simulink model "RCkolo"  (R2015a)
settings: Solver=ode45  StartTime=0.0  StopTime=0.1  MaxStep=10e-6  RelTol=1e-3
values from neighbouring files (symbols this model uses):
  C = 1000e-6    (= 0.001)    [MfajlRCkolo.m]
  R = 5    [MfajlRCkolo.m]
  V = 15    [MfajlRCkolo.m]
libraries: powerlib x6
settings Model: Creator=BLAGI  LastModifiedBy=BLAGI

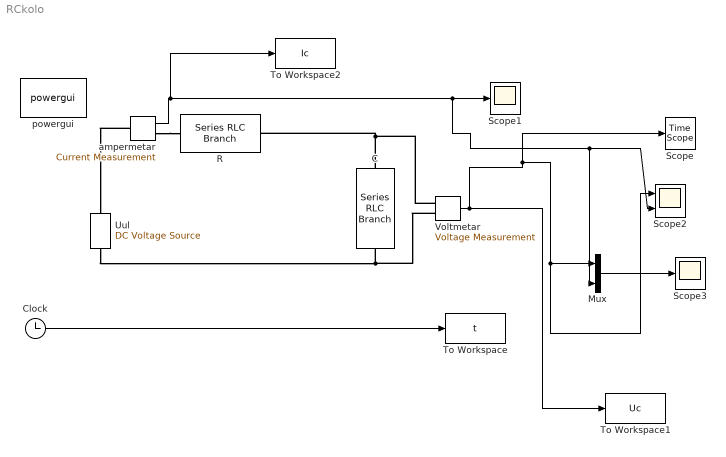
== system RCkolo ==
  C : powerlib/Elements/Series RLC Branch  LConnTagsString=__new0  RConnTagsString=__new0  BranchType=C  Resistance=5  Inductance=1e-3  SetiL0=off  InitialCurrent=0  Capacitance=C  Setx0=on  InitialVoltage=0  Measurements=None
  Clock : Clock
  Mux : Mux  Inputs=2
  R : powerlib/Elements/Series RLC Branch  LConnTagsString=__new0  RConnTagsString=__new0  BranchType=R  Resistance=R  Inductance=1e-3  SetiL0=off  InitialCurrent=0  Capacitance=1e-6  Setx0=off  InitialVoltage=0  Measurements=None
  Scope : TimeScope
  Scope1 : Scope
  Scope2 : Scope  NumInputPorts=2
      settings: YMin=-5~-5  YMax=5~5  SaveName=ScopeData2
  Scope3 : Scope
      settings: SaveName=ScopeData3
  To Workspace : ToWorkspace  VariableName=t  SampleTime=-1
  To Workspace1 : ToWorkspace  VariableName=Uc  SampleTime=-1
  To Workspace2 : ToWorkspace  VariableName=Ic  SampleTime=-1
  Uul : powerlib/Electrical Sources/DC Voltage Source  Amplitude=V  Measurements=None
  Voltmetar : powerlib/Measurements/Voltage Measurement  PhasorSimulation=off  OutputType=Complex  PSBequivalent=0
  ampermetar : powerlib/Measurements/Current Measurement  PhasorSimulation=off  OutputType=Complex  PSBequivalent=0
  powergui : powerlib/powergui  Priority=1  SimulationMode=Continuous  SolverType=Tustin/Backward Euler (TBE)  SampleTime=50e-6  frequency=60  SPID=off  DisableSnubberDevices=off  DisableRonSwitches=off  DisableVfSwitches=off  SwTol=0  DisplayEquations=off  Interpol=off  methode=off  Ts=100  FunctionMessages=off  echomessages=off  HookPort=off  EnableUseOfTLC=off  x0status=blocks  frequencyindice=0  Pbase=100e6  ErrMax=1e-4  Iterations=50  UnitsV=kV  UnitsW=MW  buscounter=0  RestoreLinks=warning  ResistiveCurrentMeasurement=off  Frange=[0:2:500]  Ylog=off  Xlog=on  ShowGrid=off  save=off  variable=ZData  structure=0  ZoomFFT=off  StartTime=0.0  cycles=1  DisplayStyle=1  fundamental=60  FreqAxis=off  MaxFrequency=1000  frequencyindicesteady=1  RmsSteady=1  display=off
  wires:
  Voltmetar/1 -> To Workspace1/1, Mux/1, Scope2/1, Scope/1
  ampermetar/1 -> To Workspace2/1, Mux/2, Scope2/2, Scope1/1
  Mux/1 -> Scope3/1
  Clock/1 -> To Workspace/1
  connections:
  Uul/LConn1 -- Voltmetar/LConn2 -- C/RConn1
  C/LConn1 -- Voltmetar/LConn1 -- R/RConn1
  ampermetar/RConn1 -- R/LConn1
  ampermetar/LConn1 -- Uul/RConn1
